simulink model "TST_CoPT_ThermDem"  (R2016b)
settings: Solver=FixedStepDiscrete  StartTime=0.0  StopTime=simTime  FixedStep=sampleTime  RelTol=1e-3
values from neighbouring files (symbols this model uses):
  testCase = 1    [initTST_CoPT_ThermDem_001.m]
libraries: simulink x4, UnitTest_Lib x2
settings Model: Creator=zhengjinyan  LastModifiedBy=zhengjinyan
settings DebuggingCC: SignalRangeChecking=error

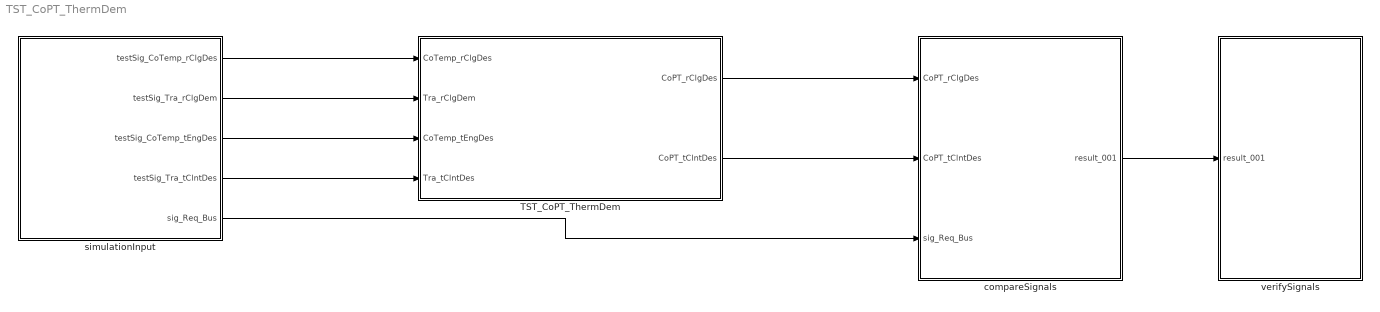
== system TST_CoPT_ThermDem ==
  TST_CoPT_ThermDem : Subsystem
  compareSignals : Subsystem
  simulationInput : Subsystem
  verifySignals : Subsystem
  wires:
  simulationInput/1(testSig_CoTemp_rClgDes) -> TST_CoPT_ThermDem/1(CoTemp_rClgDes)
  simulationInput/2(testSig_Tra_rClgDem) -> TST_CoPT_ThermDem/2(Tra_rClgDem)
  simulationInput/3(testSig_CoTemp_tEngDes) -> TST_CoPT_ThermDem/3(CoTemp_tEngDes)
  simulationInput/4(testSig_Tra_tClntDes) -> TST_CoPT_ThermDem/4(Tra_tClntDes)
  TST_CoPT_ThermDem/1(CoPT_rClgDes) -> compareSignals/1(CoPT_rClgDes)
  TST_CoPT_ThermDem/2(CoPT_tClntDes) -> compareSignals/2(CoPT_tClntDes)
  simulationInput/5(sig_Req_Bus) -> compareSignals/3(sig_Req_Bus)
  compareSignals/1(result_001) -> verifySignals/1(result_001)

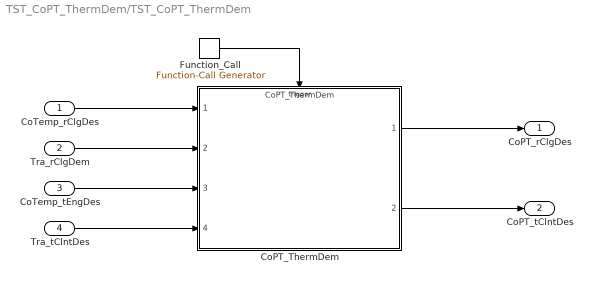
== system TST_CoPT_ThermDem/TST_CoPT_ThermDem ==
  CoTemp_rClgDes : Inport
  Tra_rClgDem : Inport  Port=2
  CoTemp_tEngDes : Inport  Port=3
  Tra_tClntDes : Inport  Port=4
  CoPT_ThermDem : ModelReference  ModelNameDialog=CoPT_ThermDem  SimulationMode=Normal  ModelReferenceVersion=1.7  TriggerPortName=function  TriggerPortTriggerType=function-call  TriggerPortStatesWhenEnabling=held
  Function_Call : simulink/Ports & Subsystems/Function-Call Generator  sample_time=sampleTime  numberOfIterations=1
  CoPT_rClgDes : Outport
  CoPT_tClntDes : Outport  Port=2
  wires:
  Function_Call/1 -> CoPT_ThermDem/Trigger
  CoTemp_rClgDes/1 -> CoPT_ThermDem/1
  Tra_rClgDem/1 -> CoPT_ThermDem/2
  CoTemp_tEngDes/1 -> CoPT_ThermDem/3
  Tra_tClntDes/1 -> CoPT_ThermDem/4
  CoPT_ThermDem/1 -> CoPT_rClgDes/1
  CoPT_ThermDem/2 -> CoPT_tClntDes/1

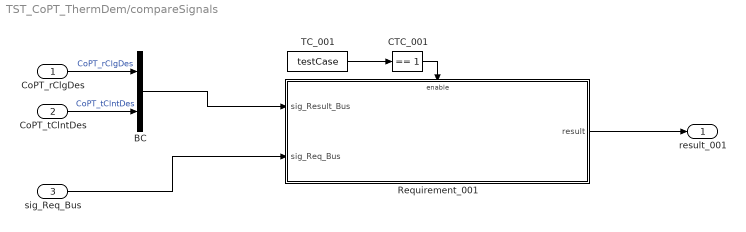
== system TST_CoPT_ThermDem/compareSignals ==
  CoPT_rClgDes : Inport
  CoPT_tClntDes : Inport  Port=2
  sig_Req_Bus : Inport  Port=3
  BC : BusCreator  Inputs=2
  CTC_001 : simulink/Logic and Bit Operations/Compare To Constant  relop===  const=1  OutDataTypeStr=boolean
  Requirement_001 : Subsystem
  TC_001 : Constant  Value=testCase
  result_001 : Outport
  wires:
  CoPT_rClgDes/1 -> BC/1  "CoPT_rClgDes"
  CoPT_tClntDes/1 -> BC/2  "CoPT_tClntDes"
  TC_001/1 -> CTC_001/1
  CTC_001/1 -> Requirement_001/Enable
  sig_Req_Bus/1 -> Requirement_001/2(sig_Req_Bus)
  BC/1 -> Requirement_001/1(sig_Result_Bus)
  Requirement_001/1(result) -> result_001/1

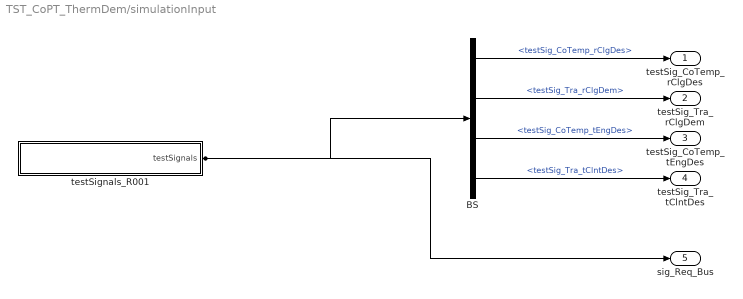
== system TST_CoPT_ThermDem/simulationInput ==
  BS : BusSelector  OutputSignals=testSig_CoTemp_rClgDes,testSig_Tra_rClgDem,testSig_CoTemp_tEngDes,testSig_Tra_tClntDes
  testSignals_R001 : Subsystem
  testSig_CoTemp_rClgDes : Outport
  testSig_Tra_rClgDem : Outport  Port=2
  testSig_CoTemp_tEngDes : Outport  Port=3
  testSig_Tra_tClntDes : Outport  Port=4
  sig_Req_Bus : Outport  Port=5
  wires:
  BS/1 -> testSig_CoTemp_rClgDes/1  "<testSig_CoTemp_rClgDes>"
  BS/2 -> testSig_Tra_rClgDem/1  "<testSig_Tra_rClgDem>"
  BS/3 -> testSig_CoTemp_tEngDes/1  "<testSig_CoTemp_tEngDes>"
  BS/4 -> testSig_Tra_tClntDes/1  "<testSig_Tra_tClntDes>"
  testSignals_R001/1(testSignals) -> BS/1, sig_Req_Bus/1

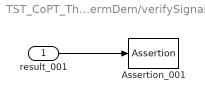
== system TST_CoPT_ThermDem/verifySignals ==
  result_001 : Inport
  Assertion_001 : Assertion  Enabled=off
  wires:
  result_001/1 -> Assertion_001/1

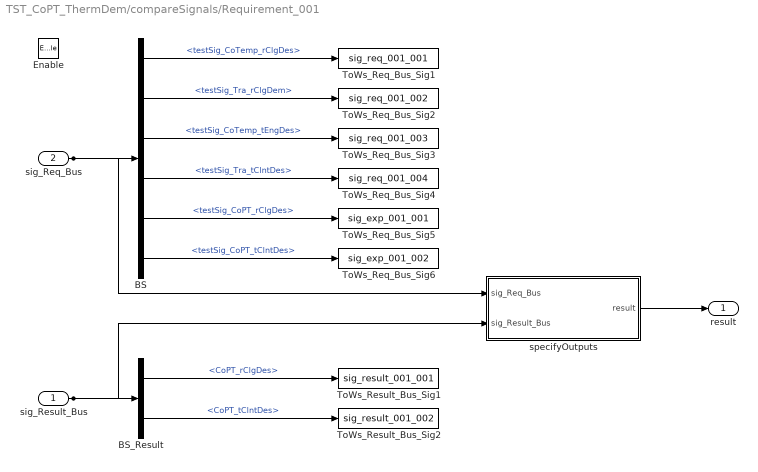
== system TST_CoPT_ThermDem/compareSignals/Requirement_001 ==
  sig_Result_Bus : Inport
  sig_Req_Bus : Inport  Port=2
  Enable : EnablePort
  BS : BusSelector  OutputSignals=testSig_CoTemp_rClgDes,testSig_Tra_rClgDem,testSig_CoTemp_tEngDes,testSig_Tra_tClntDes,testSig_CoPT_rClgDes,testSig_CoPT_tClntDes
  BS_Result : BusSelector  OutputSignals=CoPT_rClgDes,CoPT_tClntDes
  ToWs_Req_Bus_Sig1 : ToWorkspace  VariableName=sig_req_001_001  SaveFormat=Structure With Time
  ToWs_Req_Bus_Sig2 : ToWorkspace  VariableName=sig_req_001_002  SaveFormat=Structure With Time
  ToWs_Req_Bus_Sig3 : ToWorkspace  VariableName=sig_req_001_003  SaveFormat=Structure With Time
  ToWs_Req_Bus_Sig4 : ToWorkspace  VariableName=sig_req_001_004  SaveFormat=Structure With Time
  ToWs_Req_Bus_Sig5 : ToWorkspace  VariableName=sig_exp_001_001  SaveFormat=Structure With Time
  ToWs_Req_Bus_Sig6 : ToWorkspace  VariableName=sig_exp_001_002  SaveFormat=Structure With Time
  ToWs_Result_Bus_Sig1 : ToWorkspace  VariableName=sig_result_001_001  SaveFormat=Structure With Time
  ToWs_Result_Bus_Sig2 : ToWorkspace  VariableName=sig_result_001_002  SaveFormat=Structure With Time
  specifyOutputs : Subsystem
  result : Outport
  wires:
  sig_Req_Bus/1 -> BS/1, specifyOutputs/1(sig_Req_Bus)
  BS/1 -> ToWs_Req_Bus_Sig1/1  "<testSig_CoTemp_rClgDes>"
  BS/2 -> ToWs_Req_Bus_Sig2/1  "<testSig_Tra_rClgDem>"
  BS/3 -> ToWs_Req_Bus_Sig3/1  "<testSig_CoTemp_tEngDes>"
  BS/4 -> ToWs_Req_Bus_Sig4/1  "<testSig_Tra_tClntDes>"
  BS/5 -> ToWs_Req_Bus_Sig5/1  "<testSig_CoPT_rClgDes>"
  BS/6 -> ToWs_Req_Bus_Sig6/1  "<testSig_CoPT_tClntDes>"
  sig_Result_Bus/1 -> BS_Result/1, specifyOutputs/2(sig_Result_Bus)
  BS_Result/1 -> ToWs_Result_Bus_Sig1/1  "<CoPT_rClgDes>"
  BS_Result/2 -> ToWs_Result_Bus_Sig2/1  "<CoPT_tClntDes>"
  specifyOutputs/1(result) -> result/1

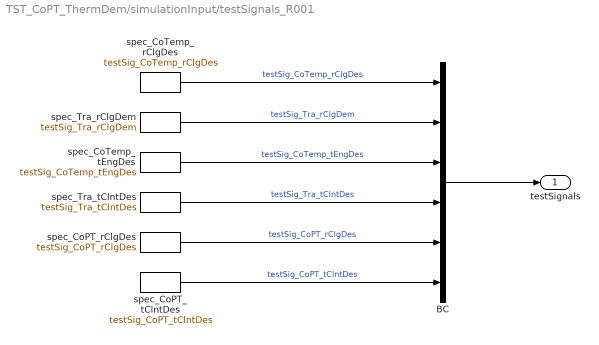
== system TST_CoPT_ThermDem/simulationInput/testSignals_R001 ==
  BC : BusCreator  Inputs=6
  spec_CoPT_rClgDes : FromWorkspace  VariableName=testSig_CoPT_rClgDes  Interpolate=off  OutputAfterFinalValue=Holding final value
  spec_CoPT_tClntDes : FromWorkspace  VariableName=testSig_CoPT_tClntDes  Interpolate=off  OutputAfterFinalValue=Holding final value
  spec_CoTemp_rClgDes : FromWorkspace  VariableName=testSig_CoTemp_rClgDes  Interpolate=off  OutputAfterFinalValue=Holding final value
  spec_CoTemp_tEngDes : FromWorkspace  VariableName=testSig_CoTemp_tEngDes  Interpolate=off  OutputAfterFinalValue=Holding final value
  spec_Tra_rClgDem : FromWorkspace  VariableName=testSig_Tra_rClgDem  Interpolate=off  OutputAfterFinalValue=Holding final value
  spec_Tra_tClntDes : FromWorkspace  VariableName=testSig_Tra_tClntDes  Interpolate=off  OutputAfterFinalValue=Holding final value
  testSignals : Outport
  wires:
  BC/1 -> testSignals/1
  spec_CoTemp_rClgDes/1 -> BC/1  "testSig_CoTemp_rClgDes"
  spec_Tra_rClgDem/1 -> BC/2  "testSig_Tra_rClgDem"
  spec_CoTemp_tEngDes/1 -> BC/3  "testSig_CoTemp_tEngDes"
  spec_Tra_tClntDes/1 -> BC/4  "testSig_Tra_tClntDes"
  spec_CoPT_rClgDes/1 -> BC/5  "testSig_CoPT_rClgDes"
  spec_CoPT_tClntDes/1 -> BC/6  "testSig_CoPT_tClntDes"

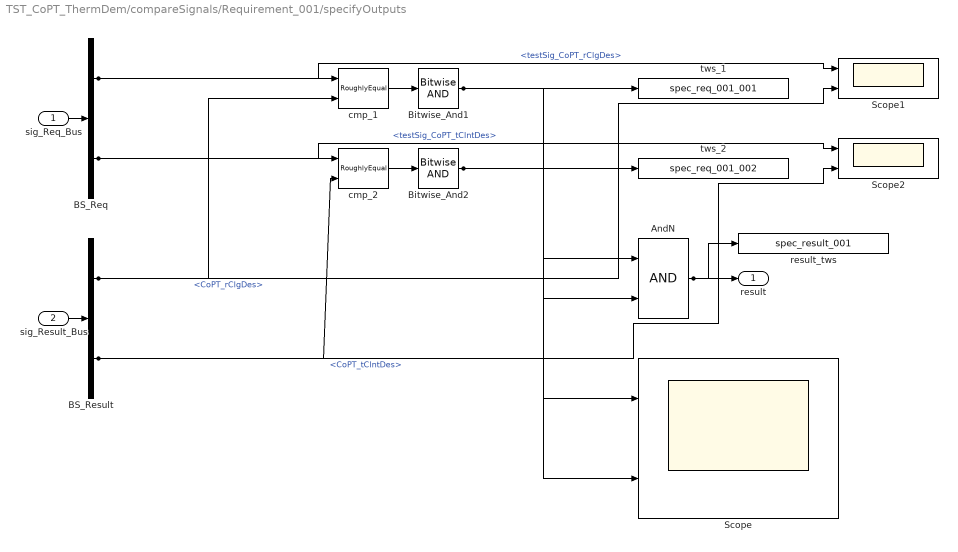
== system TST_CoPT_ThermDem/compareSignals/Requirement_001/specifyOutputs ==
  sig_Req_Bus : Inport
  sig_Result_Bus : Inport  Port=2
  AndN : Logic
  BS_Req : BusSelector  OutputSignals=testSig_CoPT_rClgDes,testSig_CoPT_tClntDes
  BS_Result : BusSelector  OutputSignals=CoPT_rClgDes,CoPT_tClntDes
  Bitwise_And1 : simulink/Logic and Bit Operations/Bitwise Operator  logicop=AND  UseBitMask=off  BitMask=bin2dec('11011001')  BitMaskRealWorld=Stored Integer
  Bitwise_And2 : simulink/Logic and Bit Operations/Bitwise Operator  logicop=AND  UseBitMask=off  BitMask=bin2dec('11011001')  BitMaskRealWorld=Stored Integer
  Scope : Scope  NumInputPorts=2
  Scope1 : Scope  NumInputPorts=2
  Scope2 : Scope  NumInputPorts=2
  cmp_1 : UnitTest_Lib/RoughlyEqual  slope=0.1
  cmp_2 : UnitTest_Lib/RoughlyEqual  slope=0.1
  result_tws : ToWorkspace  VariableName=spec_result_001
  tws_1 : ToWorkspace  VariableName=spec_req_001_001
  tws_2 : ToWorkspace  VariableName=spec_req_001_002
  result : Outport
  wires:
  sig_Req_Bus/1 -> BS_Req/1
  sig_Result_Bus/1 -> BS_Result/1
  AndN/1 -> result/1, result_tws/1
  BS_Req/1 -> cmp_1/1, Scope1/1  "<testSig_CoPT_rClgDes>"
  BS_Result/1 -> cmp_1/2, Scope1/2  "<CoPT_rClgDes>"
  cmp_1/1 -> Bitwise_And1/1
  Bitwise_And1/1 -> tws_1/1, AndN/1, Scope/1
  BS_Req/2 -> cmp_2/1, Scope2/1  "<testSig_CoPT_tClntDes>"
  BS_Result/2 -> cmp_2/2, Scope2/2  "<CoPT_tClntDes>"
  cmp_2/1 -> Bitwise_And2/1
  Bitwise_And2/1 -> tws_2/1, AndN/2, Scope/2
